simulink model "projectSimulinkpart3"  (R2022a)
settings: Solver=VariableStepAuto  StartTime=0.0  StopTime=10.0  RelTol=1e-3
values from neighbouring files (symbols this model uses):
  Caf = d(1)    [SysODE.m]    (also in scriptMatlabPart3.m = 10)
  Caf_step = 0    [scriptMatlabPart3.m]
  Caf_t_step = 1    [scriptMatlabPart3.m]
  Cb0 = k1*V*Ca0/(q_nom+k2*V)    (= 1.98710846154)    [scriptMatlabPart3.m]
  Cb_set = 1.1*Cb0    (= 2.18581930769)    [scriptMatlabPart3.m]
  k1 = d(2)    [SysODE.m]    (also in scriptMatlabPart3.m = 4.16666666667)
  k1_step = 0    [scriptMatlabPart3.m]
  k1_t_step = 1    [scriptMatlabPart3.m]
  k2 = d(3)    [SysODE.m]    (also in scriptMatlabPart3.m = 1.66666666667)
  k2_step = 1.1    [scriptMatlabPart3.m]
  k2_t_step = 1    [scriptMatlabPart3.m]
  k3 = p(2)    [SysODE.m]    (also in scriptMatlabPart3.m = 0.166666666667)
  Nd = 3    [scriptMatlabPart3.m]
  Np = 2    [scriptMatlabPart3.m]
  Nu = 1    [scriptMatlabPart3.m]
  Ny = Nx    (= 2)    [scriptMatlabPart3.m]
  q_nom = 5000    [scriptMatlabPart3.m]
  V = p(1)    [SysODE.m]    (also in scriptMatlabPart3.m = 10000)
  x0 = [Ca0; Cb0]    [scriptMatlabPart3.m]
undefined symbols (not defined in the file or in its folder): SysODE
libraries: slpidlib x1
settings Model: Creator=kirat  LastModifiedBy=andre

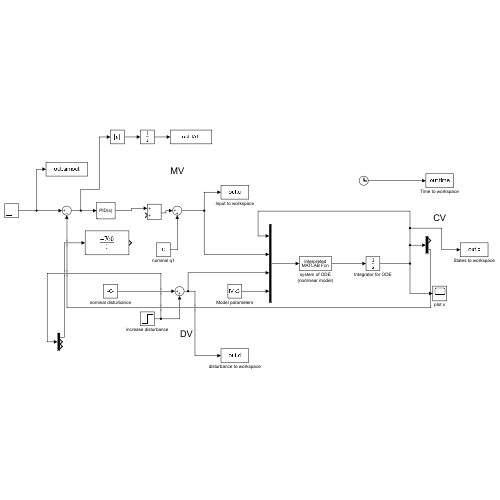
[thumbnail: Simulink's stored preview of the top-level diagram]
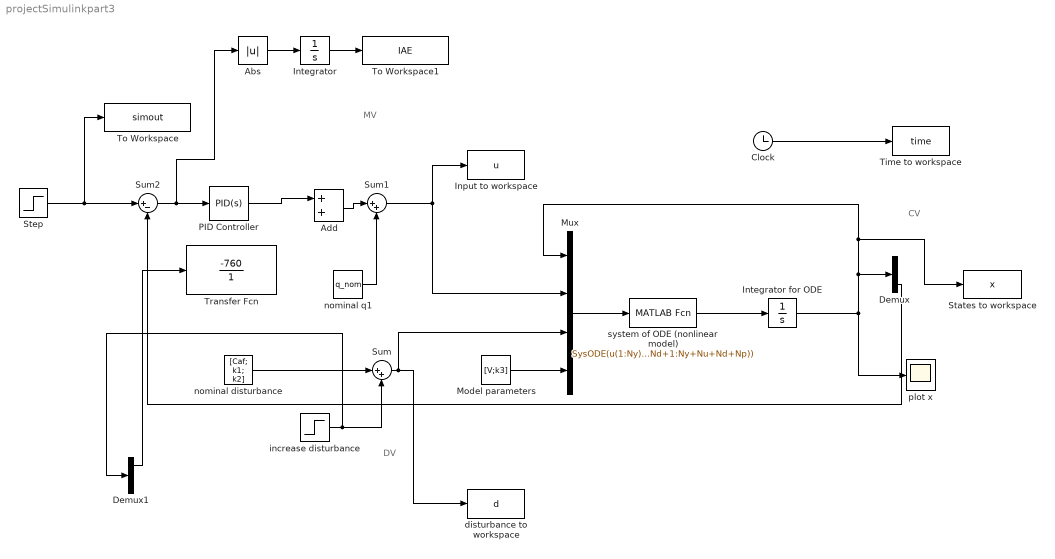
== system projectSimulinkpart3 ==
  note: DV
  note: MV
  note: CV
  Abs : Abs  SaturateOnIntegerOverflow=off
  Add : Sum
  Clock : Clock
  Demux : Demux  Outputs=2
  Demux1 : Demux  Outputs=3
  Input to workspace : ToWorkspace  VariableName=u  SampleTime=-1
  Integrator : Integrator
  Integrator for ODE : Integrator  InitialCondition=x0'
  Model parameters : Constant  Value=[V;k3]
  Mux : Mux
  PID Controller : slpidlib/PID Controller  Controller=PID  Form=Parallel  TimeDomain=Continuous-time  UseExternalTs=off  SampleTime=-1  IntegratorMethod=Forward Euler  FilterMethod=Forward Euler  ControllerParametersSource=internal  P=5909  I=11445  UseKiTs=off  D=0  N=100  UseFilter=on  TunerSelectOption=Transfer Function Based (PID Tuner App)  InitialConditionSource=internal  InitialConditionForIntegrator=0  InitialConditionForFilter=0  DifferentiatorICPrevScaledInput=0  ExternalReset=none  TrackingMode=off  Kt=1  LimitOutput=off  SatLimitsSource=internal  UpperSaturationLimit=inf  LowerSaturationLimit=-inf  LinearizeAsGain=on  AntiWindupMode=none  Kb=1  POutMin=[]  POutMax=[]  IOutMin=[]  IOutMax=[]  DOutMin=[]  DOutMax=[]  NOutMin=[]  NOutMax=[]  SumOutMin=[]  SumOutMax=[]  SaturationOutMin=[]  SaturationOutMax=[]  PParamMin=[]  PParamMax=[]  IParamMin=[]  IParamMax=[]  DParamMin=[]  DParamMax=[]  NParamMin=[]  NParamMax=[]  KbParamMin=[]  KbParamMax=[]  KtParamMin=[]  KtParamMax=[]  KbOutMin=[]  KbOutMax=[]  KtOutMin=[]  KtOutMax=[]  IntegratorOutMin=[]  IntegratorOutMax=[]  FilterOutMin=[]  FilterOutMax=[]  SumI1OutMin=[]  SumI1OutMax=[]  SumI2OutMin=[]  SumI2OutMax=[]  SumI3OutMin=[]  SumI3OutMax=[]  SumI4OutMin=[]  SumI4OutMax=[]  SumDOutMin=[]  SumDOutMax=[]  DifferentiatorOutMin=[]  DifferentiatorOutMax=[]  FilterDiffOutCoefMin=[]  FilterDiffOutCoefMax=[]  ReciprocalOutMin=[]  ReciprocalOutMax=[]  SumDenOutMin=[]  SumDenOutMax=[]  SumNumOutMin=[]  SumNumOutMax=[]  DivideOutMin=[]  DivideOutMax=[]  UdiffTsProdOutMin=[]  UdiffTsProdOutMax=[]  NTsProdOutMin=[]  NTsProdOutMax=[]  UintegralTsProdOutMin=[]  UintegralTsProdOutMax=[]  UngainTsProdOutMin=[]  UngainTsProdOutMax=[]  IntegratorContinuousStateAttributes=''  IntegratorStateMustResolveToSignalObject=off  IntegratorRTWStateStorageClass=Auto  FilterContinuousStateAttributes=''  FilterStateMustResolveToSignalObject=off  FilterRTWStateStorageClass=Auto  ParallelPVariant=InternalParameters  IdealPVariant=Disabled  IVariant=InternalParameters  DVariant=InternalParameters  IntegratorVariant=Continuous  SatVariant=Disabled  AWVariant=Passthrough  PCopyVariant=Disabled  TRVariant=Disabled  FdbkBlocksVariant=Forward  IdealPFdbkVariant=Disabled  SatFdbkVariant=Disabled  DerivativeFilterVariant=ContFilter  NVariant=InternalParameters  NCopyVariant=Disabled  FilterICVariant=InternalICsFilter  IntegratorICVariant=InternalICs  ExternalResetVariant=Disabled  TRSumVariant=Passthrough  SumFdbkVariant=Disabled  SumVariant=Sum_PID  TsampFilterVariant=InternalTs  TsampNgainVariant=Passthrough  TsampIntegralVariant=Passthrough  ExternalSaturationOutDataTypeStr=Inherit: Same as second input  aMode=0
  States to workspace : ToWorkspace  VariableName=x  SampleTime=-1
  Step : Step  Before=Cb0  After=Cb_set  SampleTime=0
  Sum : Sum  Inputs=|++
  Sum1 : Sum  Inputs=|++
  Sum2 : Sum  Inputs=|+-
  Time to workspace : ToWorkspace  VariableName=time  SampleTime=-1
  To Workspace : ToWorkspace  VariableName=simout  SaveFormat=Timeseries  SampleTime=-1
  To Workspace1 : ToWorkspace  VariableName=IAE  SampleTime=-1
  Transfer Fcn : TransferFcn  Numerator=[-760]  Denominator=[1]
  disturbance to workspace : ToWorkspace  VariableName=d  SampleTime=-1
  increase disturbance : Step  Time=[Caf_t_step; k1_t_step; k2_t_step]  Before=[0; 0; 0]  After=[Caf_step;k1_step; k2_step];  SampleTime=0
  nominal disturbance : Constant  Value=[Caf; k1; k2]
  nominal q1 : Constant  Value=q_nom
  plot x : Scope
  system of ODE (nonlinear model) : MATLABFcn  MATLABFcn=SysODE(u(1:Ny),u(Ny+1:Ny+Nu),u(Ny+Nu+1:Ny+Nu+Nd),u(Ny+Nu+Nd+1:Ny+Nu+Nd+Np))  OutputDimensions=Ny  Output1D=off
  wires:
  increase disturbance/1 -> Demux1/1, Sum/2
  Clock/1 -> Time to workspace/1
  system of ODE (nonlinear model)/1 -> Integrator for ODE/1
  Mux/1 -> system of ODE (nonlinear model)/1
  Sum1/1 -> Input to workspace/1, Mux/2
  nominal q1/1 -> Sum1/2
  Model parameters/1 -> Mux/4
  nominal disturbance/1 -> Sum/1
  Sum2/1 -> Abs/1, PID Controller/1
  Integrator for ODE/1 -> plot x/1, Demux/1, States to workspace/1, Mux/1
  Demux/2 -> Sum2/2
  Step/1 -> To Workspace/1, Sum2/1
  Sum/1 -> disturbance to workspace/1, Mux/3
  PID Controller/1 -> Add/1
  Demux1/1 -> Transfer Fcn/1
  Add/1 -> Sum1/1
  Abs/1 -> Integrator/1
  Integrator/1 -> To Workspace1/1
